simulink model "CaseStudyI_9_Bus"  (R2020a)
settings: Solver=FixedStepAuto  StartTime=0.0  StopTime=Tend  FixedStep=T_s_power  MaxStep=5.0E-5  RelTol=1e-3
values from neighbouring files (symbols this model uses):
  B_s46 = b_s46*Cb    (= 9.5071761847e-07)    [Data_CaseStudyI.m]    (also in Data_CaseStudyII.m; Data_InitialSystem.m)
  B_s54 = b_s54*Cb    (= 1.05902722057e-06)    [Data_CaseStudyI.m]    (also in Data_CaseStudyII.m; Data_InitialSystem.m)
  B_s69 = b_s69*Cb    (= 2.15415764185e-06)    [Data_CaseStudyI.m]    (also in Data_CaseStudyII.m; Data_InitialSystem.m)
  B_s75 = b_s75*Cb    (= 1.84126323577e-06)    [Data_CaseStudyI.m]    (also in Data_CaseStudyII.m; Data_InitialSystem.m)
  B_s87 = b_s87*Cb    (= 8.96562817417e-07)    [Data_CaseStudyI.m]    (also in Data_CaseStudyII.m; Data_InitialSystem.m)
  B_s98 = b_s98*Cb    (= 1.25759482443e-06)    [Data_CaseStudyI.m]    (also in Data_CaseStudyII.m; Data_InitialSystem.m)
  C_dc_DVPP_1_2 = 0.008*(n_DVPP_1_2)    (= 0.8)    [Data_CaseStudyI.m]    (also in Data_CaseStudyII.m)
  C_dc_DVPP_1_3 = 0.008*(n_DVPP_1_3)    (= 0.4)    [Data_CaseStudyI.m]    (also in Data_CaseStudyII.m)
  fb = 50    [Data_CaseStudyI.m]    (also in Data_CaseStudyII.m; Data_InitialSystem.m)
  HGov_dyn = HGov_delay*H_tr_droop    [Data_CaseStudyI.m]    (also in Data_CaseStudyII.m; Data_InitialSystem.m)
  HTurb_tot = H_water_way    [Data_CaseStudyI.m]    (also in Data_CaseStudyII.m; Data_InitialSystem.m)
  I_m_DVPP_1_2 = 2/3*Sb_DVPP_1_2/V_m_DVPP_1_2    [Data_CaseStudyI.m]    (also in Data_CaseStudyII.m)
  I_m_DVPP_1_3 = 2/3*Sb_DVPP_1_3/V_m_DVPP_1_3    [Data_CaseStudyI.m]    (also in Data_CaseStudyII.m)
  i_star_max = 1.3    [Data_CaseStudyI.m]    (also in Data_CaseStudyII.m)
  iabc_DVPP_1_2_0 = T0*idq0_DVPP_1_2    [Data_CaseStudyI.m]    (also in Data_CaseStudyII.m)
  iabc_DVPP_1_3_0 = T0*idq0_DVPP_1_3    [Data_CaseStudyI.m]    (also in Data_CaseStudyII.m)
  K2_DVPP_1 = [-0.0221795494247 -1.60799665656 0.160449825826 -2.94803557381 -11.8081988371 -9.75170960256 0.00463021906909 -49.1667298155]    [ControlGains_DVPP1.mat]
  K3_DVPP_1 = [-0.0591512752956 -1.61493903379 -27.2946107927 -16.2119211358 -14.3657419818 2.05688388773 -2.27328406162 0.146700393037 -150.920793597]    [ControlGains_DVPP1.mat]
  k_dc_DVPP_1_2 = eta_DVPP_1_2/(Vdc_n_DVPP_1_2*m_p_DVPP_1_2)    [Data_CaseStudyI.m]    (also in Data_CaseStudyII.m)
  k_dc_DVPP_1_3 = eta_DVPP_1_3/(Vdc_n_DVPP_1_3*m_p_DVPP_1_3)    [Data_CaseStudyI.m]    (also in Data_CaseStudyII.m)
  ki_i_pu = 1.19    [Data_CaseStudyI.m]    (also in Data_CaseStudyII.m)
  ki_pll = 1700    [Data_CaseStudyI.m]    (also in Data_CaseStudyII.m)
  ki_q_pu = 0.005    [Data_CaseStudyI.m]    (also in Data_CaseStudyII.m)
  kp_i_pu = 0.73    [Data_CaseStudyI.m]    (also in Data_CaseStudyII.m)
  kp_pll = 150    [Data_CaseStudyI.m]    (also in Data_CaseStudyII.m)
  kp_q_pu = 0.05    [Data_CaseStudyI.m]    (also in Data_CaseStudyII.m)
  L1_DVPP_1_2_pu = 0.0186/m_DVPP_1_2    (= 0.000372)    [Data_CaseStudyI.m]    (also in Data_CaseStudyII.m)
  L1_DVPP_1_3_pu = 0.0186/m_DVPP_1_3    (= 0.000744)    [Data_CaseStudyI.m]    (also in Data_CaseStudyII.m)
  l1_MVHV1 = 0    [Data_CaseStudyI.m]    (also in Data_CaseStudyII.m; Data_InitialSystem.m)
  l1_MVHV2 = 0    [Data_CaseStudyI.m]    (also in Data_CaseStudyII.m; Data_InitialSystem.m)
  l1_MVHV3 = 0    [Data_CaseStudyI.m]    (also in Data_CaseStudyII.m; Data_InitialSystem.m)
  L2_DVPP_1_2_pu = L1_DVPP_1_2_pu    (= 0.000372)    [Data_CaseStudyI.m]    (also in Data_CaseStudyII.m)
  L2_DVPP_1_3_pu = L1_DVPP_1_3_pu    (= 0.000744)    [Data_CaseStudyI.m]    (also in Data_CaseStudyII.m)
  l2_MVHV1 = l_s14    (= 0.0576)    [Data_CaseStudyI.m]    (also in Data_CaseStudyII.m; Data_InitialSystem.m)
  l2_MVHV2 = l_s72    (= 0.0625)    [Data_CaseStudyI.m]    (also in Data_CaseStudyII.m; Data_InitialSystem.m)
  l2_MVHV3 = l_s39    (= 0.0586)    [Data_CaseStudyI.m]    (also in Data_CaseStudyII.m; Data_InitialSystem.m)
  l_f_DVPP_1_2 = L_f_DVPP_1_2*w_b/Zb_DVPP_1_2    [Data_CaseStudyI.m]    (also in Data_CaseStudyII.m)
  L_f_DVPP_1_2 = (1/(n_DVPP_1_2))*600*10^-6    (= 6e-06)    [Data_CaseStudyI.m]    (also in Data_CaseStudyII.m)
  l_f_DVPP_1_3 = L_f_DVPP_1_3*w_b/Zb_DVPP_1_3    [Data_CaseStudyI.m]    (also in Data_CaseStudyII.m)
  L_f_DVPP_1_3 = (1/(n_DVPP_1_3))*600*10^-6    (= 1.2e-05)    [Data_CaseStudyI.m]    (also in Data_CaseStudyII.m)
  L_s46 = l_s46*Lb    (= 0.154915055408)    [Data_CaseStudyI.m]    (also in Data_CaseStudyII.m; Data_InitialSystem.m)
  L_s54 = l_s54*Lb    (= 0.143128040323)    [Data_CaseStudyI.m]    (also in Data_CaseStudyII.m; Data_InitialSystem.m)
  L_s69 = l_s69*Lb    (= 0.286256080645)    [Data_CaseStudyI.m]    (also in Data_CaseStudyII.m; Data_InitialSystem.m)
  L_s75 = l_s75*Lb    (= 0.271101346964)    [Data_CaseStudyI.m]    (also in Data_CaseStudyII.m; Data_InitialSystem.m)
  L_s87 = l_s87*Lb    (= 0.12123786945)    [Data_CaseStudyI.m]    (also in Data_CaseStudyII.m; Data_InitialSystem.m)
  L_s98 = l_s98*Lb    (= 0.16973301723)    [Data_CaseStudyI.m]    (also in Data_CaseStudyII.m; Data_InitialSystem.m)
  P_L = pL*Sb    (= 300000000)    [Data_CaseStudyI.m]    (also in Data_CaseStudyII.m; Data_InitialSystem.m)
  p_set_bus1 = P_set_bus1/SbSG1    (= 0.731707317073)    [Data_CaseStudyI.m]    (also in Data_CaseStudyII.m; Data_InitialSystem.m)
  p_set_bus2 = P_set_bus2/SbSG2    (= 0.756707317073)    [Data_CaseStudyI.m]    (also in Data_CaseStudyII.m; Data_InitialSystem.m)
  p_set_bus3 = P_set_bus3/SbSG3    (= 0.731707317073)    [Data_CaseStudyI.m]    (also in Data_CaseStudyII.m; Data_InitialSystem.m)
  pset_DVPP_1_1 = P_set_bus1/SbSG1    (= 0.731707317073)    [Data_CaseStudyI.m]    (also in Data_CaseStudyII.m)
  pset_DVPP_1_2 = 0    [Data_CaseStudyI.m]    (also in Data_CaseStudyII.m)
  pset_DVPP_1_3 = 0    [Data_CaseStudyI.m]    (also in Data_CaseStudyII.m)
  Q_L = qL*Sb    (= 82500000)    [Data_CaseStudyI.m]    (also in Data_CaseStudyII.m; Data_InitialSystem.m)
  qset_DVPP_1_2 = 0    [Data_CaseStudyI.m]    (also in Data_CaseStudyII.m)
  qset_DVPP_1_3 = 0    [Data_CaseStudyI.m]    (also in Data_CaseStudyII.m)
  R1_DVPP_1_2_pu = 0.00734/m_DVPP_1_2    (= 0.0001468)    [Data_CaseStudyI.m]    (also in Data_CaseStudyII.m)
  R1_DVPP_1_3_pu = 0.00734/m_DVPP_1_3    (= 0.0002936)    [Data_CaseStudyI.m]    (also in Data_CaseStudyII.m)
  r1_MVHV1 = 1e-6    (= 1e-06)    [Data_CaseStudyI.m]    (also in Data_CaseStudyII.m; Data_InitialSystem.m)
  r1_MVHV2 = 1e-6    (= 1e-06)    [Data_CaseStudyI.m]    (also in Data_CaseStudyII.m; Data_InitialSystem.m)
  r1_MVHV3 = 1e-6    (= 1e-06)    [Data_CaseStudyI.m]    (also in Data_CaseStudyII.m; Data_InitialSystem.m)
  R2_DVPP_1_2_pu = R1_DVPP_1_2_pu    (= 0.0001468)    [Data_CaseStudyI.m]    (also in Data_CaseStudyII.m)
  R2_DVPP_1_3_pu = R1_DVPP_1_3_pu    (= 0.0002936)    [Data_CaseStudyI.m]    (also in Data_CaseStudyII.m)
  r2_MVHV1 = 1e-6    (= 1e-06)    [Data_CaseStudyI.m]    (also in Data_CaseStudyII.m; Data_InitialSystem.m)
  r2_MVHV2 = 1e-6    (= 1e-06)    [Data_CaseStudyI.m]    (also in Data_CaseStudyII.m; Data_InitialSystem.m)
  r2_MVHV3 = 1e-6    (= 1e-06)    [Data_CaseStudyI.m]    (also in Data_CaseStudyII.m; Data_InitialSystem.m)
  R_dc_DVPP_1_2 = (Vdc_n_DVPP_1_2/(0.05*(Sb_DVPP_1_2)/Vdc_n_DVPP_1_2))    [Data_CaseStudyI.m]    (also in Data_CaseStudyII.m)
  R_dc_DVPP_1_3 = (Vdc_n_DVPP_1_3/(0.05*(Sb_DVPP_1_3)/Vdc_n_DVPP_1_3))    [Data_CaseStudyI.m]    (also in Data_CaseStudyII.m)
  r_f_DVPP_1_2 = R_f_DVPP_1_2/Zb_DVPP_1_2    [Data_CaseStudyI.m]    (also in Data_CaseStudyII.m)
  R_f_DVPP_1_2 = 0.02/n_DVPP_1_2    (= 0.0002)    [Data_CaseStudyI.m]    (also in Data_CaseStudyII.m)
  r_f_DVPP_1_3 = R_f_DVPP_1_3/Zb_DVPP_1_3    [Data_CaseStudyI.m]    (also in Data_CaseStudyII.m)
  R_f_DVPP_1_3 = 0.02/n_DVPP_1_3    (= 0.0004)    [Data_CaseStudyI.m]    (also in Data_CaseStudyII.m)
  R_s46 = r_s46*Zb    (= 8.993)    [Data_CaseStudyI.m]    (also in Data_CaseStudyII.m; Data_InitialSystem.m)
  R_s54 = r_s54*Zb    (= 5.29)    [Data_CaseStudyI.m]    (also in Data_CaseStudyII.m; Data_InitialSystem.m)
  R_s69 = r_s69*Zb    (= 20.631)    [Data_CaseStudyI.m]    (also in Data_CaseStudyII.m; Data_InitialSystem.m)
  R_s75 = r_s75*Zb    (= 16.928)    [Data_CaseStudyI.m]    (also in Data_CaseStudyII.m; Data_InitialSystem.m)
  R_s87 = r_s87*Zb    (= 4.4965)    [Data_CaseStudyI.m]    (also in Data_CaseStudyII.m; Data_InitialSystem.m)
  R_s98 = r_s98*Zb    (= 6.2951)    [Data_CaseStudyI.m]    (also in Data_CaseStudyII.m; Data_InitialSystem.m)
  ReferenceSS2_DVPP_1 = ss(M2T_des_DVPP_1,'minimal')    [Data_CaseStudyI.m]    (also in Data_CaseStudyII.m)
  ReferenceSS3_DVPP_1 = ss(M3T_des_DVPP_1,'minimal')    [Data_CaseStudyI.m]    (also in Data_CaseStudyII.m)
  Rg = 0.03    [Data_CaseStudyI.m]    (also in Data_CaseStudyII.m; Data_InitialSystem.m)
  Sb = 100*10^6    (= 100000000)    [Data_CaseStudyI.m]    (also in Data_CaseStudyII.m; Data_InitialSystem.m)
  Sb_DVPP_1_2 = r_b1*100*10^6*cDVPP_1_2    (= 50000000)    [Data_CaseStudyI.m]    (also in Data_CaseStudyII.m)
  Sb_DVPP_1_3 = r_b1*100*10^6*cDVPP_1_3    (= 25000000)    [Data_CaseStudyI.m]    (also in Data_CaseStudyII.m)
  SbSG1 = r_b1*100*10^6    (= 250000000)    [Data_CaseStudyI.m]    (also in Data_CaseStudyII.m; Data_InitialSystem.m)
  SbSG2 = r_b2*100*10^6    (= 96000000)    [Data_CaseStudyI.m]    (also in Data_CaseStudyII.m; Data_InitialSystem.m)
  SbSG3 = r_b3*100*10^6    (= 64000000)    [Data_CaseStudyI.m]    (also in Data_CaseStudyII.m; Data_InitialSystem.m)
  SGov_dyn = tf([1],[Tg 1])    [Data_CaseStudyI.m]    (also in Data_CaseStudyII.m; Data_InitialSystem.m)
  St_MVHV1 = Sb    (= 100000000)    [Data_CaseStudyI.m]    (also in Data_CaseStudyII.m; Data_InitialSystem.m)
  St_MVHV2 = Sb    (= 100000000)    [Data_CaseStudyI.m]    (also in Data_CaseStudyII.m; Data_InitialSystem.m)
  St_MVHV3 = Sb    (= 100000000)    [Data_CaseStudyI.m]    (also in Data_CaseStudyII.m; Data_InitialSystem.m)
  St_MVLV_DVPP_1_2 = St*m_DVPP_1_2    (= 50000000)    [Data_CaseStudyI.m]    (also in Data_CaseStudyII.m)
  St_MVLV_DVPP_1_3 = St*m_DVPP_1_3    (= 25000000)    [Data_CaseStudyI.m]    (also in Data_CaseStudyII.m)
  STurb_reheat = STurb_ch*STurb_rh    [Data_CaseStudyI.m]    (also in Data_CaseStudyII.m; Data_InitialSystem.m)
  T_load_b3 = 2010    [Data_CaseStudyI.m]    (also in Data_CaseStudyII.m = 1010)
  T_load_b6 = 1010    [Data_CaseStudyI.m]    (also in Data_InitialSystem.m)
  T_s_power = 1e-4    (= 0.0001)    [Data_CaseStudyI.m]    (also in Data_CaseStudyII.m; Data_InitialSystem.m)
  tau_dc_DVPP_1_2 = 0.2    [Data_CaseStudyI.m]    (also in Data_CaseStudyII.m)
  tau_dc_DVPP_1_3 = 0.01    [Data_CaseStudyI.m]    (also in Data_CaseStudyII.m)
  V_m_DVPP_1_2 = VbLV_DVPP_1_2*sqrt(2/3)    [Data_CaseStudyI.m]    (also in Data_CaseStudyII.m)
  V_m_DVPP_1_3 = VbLV_DVPP_1_3*sqrt(2/3)    [Data_CaseStudyI.m]    (also in Data_CaseStudyII.m)
  vabc_DVPP_1_2_0_pu = T0*vdq0_DVPP_1_2_0/V_m_DVPP_1_2    [Data_CaseStudyI.m]    (also in Data_CaseStudyII.m)
  vabc_DVPP_1_3_0_pu = T0*vdq0_DVPP_1_3_0/V_m_DVPP_1_3    [Data_CaseStudyI.m]    (also in Data_CaseStudyII.m)
  VbHV = 230*10^3    (= 230000)    [Data_CaseStudyI.m]    (also in Data_CaseStudyII.m; Data_InitialSystem.m)
  VbLV_DVPP_1_2 = 10^3    (= 1000)    [Data_CaseStudyI.m]    (also in Data_CaseStudyII.m)
  VbLV_DVPP_1_3 = 10^3    (= 1000)    [Data_CaseStudyI.m]    (also in Data_CaseStudyII.m)
  VbMV1 = 16.5*10^3    (= 16500)    [Data_CaseStudyI.m]    (also in Data_CaseStudyII.m; Data_InitialSystem.m)
  VbMV2 = 18.0*10^3    (= 18000)    [Data_CaseStudyI.m]    (also in Data_CaseStudyII.m; Data_InitialSystem.m)
  VbMV3 = 13.8*10^3    (= 13800)    [Data_CaseStudyI.m]    (also in Data_CaseStudyII.m; Data_InitialSystem.m)
  vd0_DVPP_1_2_pu = vd0_DVPP_1_2/V_m_DVPP_1_2    [Data_CaseStudyI.m]    (also in Data_CaseStudyII.m)
  vd0_DVPP_1_3_pu = vd0_DVPP_1_3/V_m_DVPP_1_3    [Data_CaseStudyI.m]    (also in Data_CaseStudyII.m)
  Vdc_n_DVPP_1_2 = 3*V_m_DVPP_1_2    [Data_CaseStudyI.m]    (also in Data_CaseStudyII.m)
  Vdc_n_DVPP_1_3 = 3*V_m_DVPP_1_3    [Data_CaseStudyI.m]    (also in Data_CaseStudyII.m)
  w_b = fb*2*pi    (= 314.159265359)    [Data_CaseStudyI.m]    (also in Data_CaseStudyII.m; Data_InitialSystem.m)
  xid0_DVPP_1_2_pu = 0    [Data_CaseStudyI.m]    (also in Data_CaseStudyII.m)
  xid0_DVPP_1_3_pu = 0    [Data_CaseStudyI.m]    (also in Data_CaseStudyII.m)
  xiq0_DVPP_1_2_pu = 0    [Data_CaseStudyI.m]    (also in Data_CaseStudyII.m)
  xiq0_DVPP_1_3_pu = 0    [Data_CaseStudyI.m]    (also in Data_CaseStudyII.m)
  xpll0_pu = w_b/(ki_pll)    (= 0.184799567858)    [Data_CaseStudyI.m]    (also in Data_CaseStudyII.m)
  xq0_DVPP_1_2_pu = xq0_DVPP_1_2/I_m_DVPP_1_2    [Data_CaseStudyI.m]    (also in Data_CaseStudyII.m)
  ... (+1 more)
undefined symbols (not defined in the file or in its folder): A, B, C, Continuous, Dd, Efd0, gcbh, i_dc, Ka, Kf, p2set, SbSM2, sps_rtmsupport, spsST1AModel, Ta, Tb, Tb1, Tc, Tc1, Tf, VA0, VAmax, VAmin, VImax, VImin, VRmax, VRmin
libraries: powerlib x73, powerlib_meascontrol x16, cstblocks x11, sps_avr x2, simulink_extras x1, simulink x1
(part 1 of 3)
settings Model: SimulationMode=accelerator  Creator=verena  LastModifiedBy=verenahaberle
settings DataIOCC: ExternalInput=getinputstruct(spec1)  FinalStateName=xFinal_c1  InitialState=xInitial_CaseStudyI  LoadInitialState=on  SaveFinalState=on  SaveOperatingPoint=on  SaveFormat=Array  ReturnWorkspaceOutputs=off  TimeSaveName=tout_c1  OutputSaveName=yout_c1  SignalLoggingName=logsout_c1  DSMLoggingName=dsmout_c1
settings OptimizationCC: BlockReduction=off
settings DebuggingCC: UnconnectedInputMsg=none  UnconnectedOutputMsg=none  UnconnectedLineMsg=none  NonCurrentReleaseOperatingPointMsg=warning

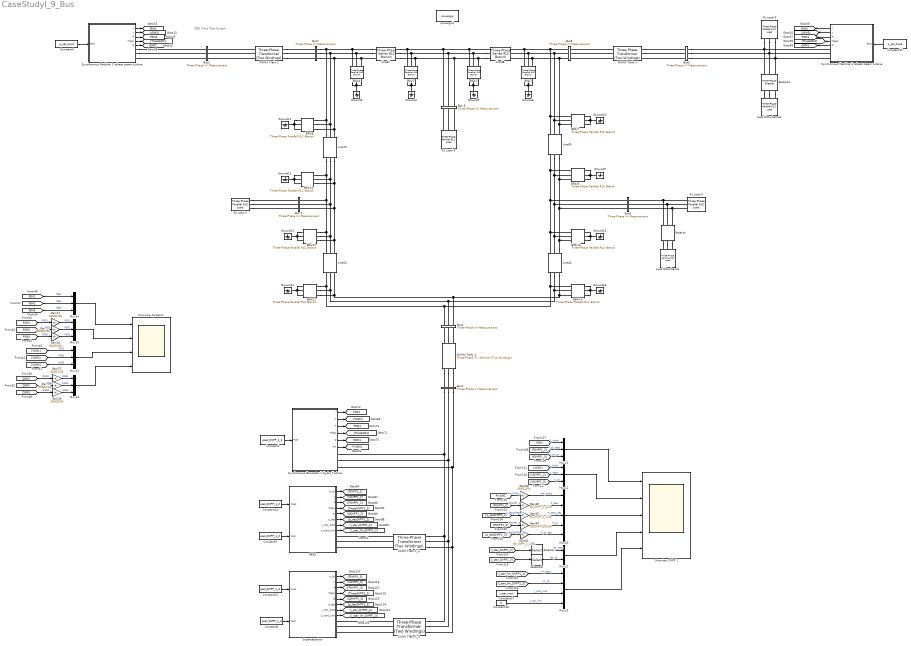
== system CaseStudyI_9_Bus ==
  note: IEEE 9-bus Test System
  B94/1 : powerlib/Elements/Three-Phase Parallel RLC Branch  LConnTagsString=A|B|C  RConnTagsString=A|B|C  BranchType=C  Resistance=1  Inductance=1e-3  Capacitance=B_s98*0.5  Measurements=None
      settings: SourceProductBaseCode=PS
  B94/10 : powerlib/Elements/Three-Phase Parallel RLC Branch  LConnTagsString=A|B|C  RConnTagsString=A|B|C  BranchType=C  Resistance=1  Inductance=1e-3  Capacitance=B_s75*0.5  Measurements=None
      settings: SourceProductBaseCode=PS
  B94/11 : powerlib/Elements/Three-Phase Parallel RLC Branch  LConnTagsString=A|B|C  RConnTagsString=A|B|C  BranchType=C  Resistance=1  Inductance=1e-3  Capacitance=B_s54*0.5  Measurements=None
      settings: SourceProductBaseCode=PS
  B94/12 : powerlib/Elements/Three-Phase Parallel RLC Branch  LConnTagsString=A|B|C  RConnTagsString=A|B|C  BranchType=C  Resistance=1  Inductance=1e-3  Capacitance=B_s54*0.5  Measurements=None
      settings: SourceProductBaseCode=PS
  B94/13 : powerlib/Elements/Three-Phase Parallel RLC Branch  LConnTagsString=A|B|C  RConnTagsString=A|B|C  BranchType=C  Resistance=1  Inductance=1e-3  Capacitance=B_s46*0.5  Measurements=None
      settings: SourceProductBaseCode=PS
  B94/14 : powerlib/Elements/Three-Phase Parallel RLC Branch  LConnTagsString=A|B|C  RConnTagsString=A|B|C  BranchType=C  Resistance=1  Inductance=1e-3  Capacitance=B_s46*0.5  Measurements=None
      settings: SourceProductBaseCode=PS
  B94/2 : powerlib/Elements/Three-Phase Parallel RLC Branch  LConnTagsString=A|B|C  RConnTagsString=A|B|C  BranchType=C  Resistance=1  Inductance=1e-3  Capacitance=B_s87*0.5  Measurements=None
      settings: SourceProductBaseCode=PS
  B94/3 : powerlib/Elements/Three-Phase Parallel RLC Branch  LConnTagsString=A|B|C  RConnTagsString=A|B|C  BranchType=C  Resistance=1  Inductance=1e-3  Capacitance=B_s98*0.5  Measurements=None
      settings: SourceProductBaseCode=PS
  B94/4 : powerlib/Elements/Three-Phase Parallel RLC Branch  LConnTagsString=A|B|C  RConnTagsString=A|B|C  BranchType=C  Resistance=1  Inductance=1e-3  Capacitance=B_s87*0.5  Measurements=None
      settings: SourceProductBaseCode=PS
  B94/7 : powerlib/Elements/Three-Phase Parallel RLC Branch  LConnTagsString=A|B|C  RConnTagsString=A|B|C  BranchType=C  Resistance=1  Inductance=1e-3  Capacitance=B_s69*0.5  Measurements=None
      settings: SourceProductBaseCode=PS
  B94/8 : powerlib/Elements/Three-Phase Parallel RLC Branch  LConnTagsString=A|B|C  RConnTagsString=A|B|C  BranchType=C  Resistance=1  Inductance=1e-3  Capacitance=B_s69*0.5  Measurements=None
      settings: SourceProductBaseCode=PS
  B94/9 : powerlib/Elements/Three-Phase Parallel RLC Branch  LConnTagsString=A|B|C  RConnTagsString=A|B|C  BranchType=C  Resistance=1  Inductance=1e-3  Capacitance=B_s75*0.5  Measurements=None
      settings: SourceProductBaseCode=PS
  BESS : Subsystem
  Breaker : powerlib/Elements/Three-Phase Breaker  InitialState=open  SwitchA=on  SwitchB=on  SwitchC=on  SwitchTimes=[T_load_b6]  External=off  BreakerResistance=0.01  SnubberResistance=1e6  SnubberCapacitance=inf  Measurements=None
  Breaker1 : powerlib/Elements/Three-Phase Breaker  InitialState=open  SwitchA=on  SwitchB=on  SwitchC=on  SwitchTimes=[T_load_b3]  External=off  BreakerResistance=0.01  SnubberResistance=1e6  SnubberCapacitance=inf  Measurements=None
  Bus 5 : powerlib/Measurements/Three-Phase V-I Measurement  VoltageMeasurement=no  SetLabelV=on  LabelV=Vabc_5  Vpu=on  VpuLL=off  CurrentMeasurement=no  SetLabelI=on  LabelI=Iabc_5  Ipu=on  Pbase=S_b  Vbase=V_b  OutputType=Complex  PhasorSimulation=off  PSBequivalent=0
  Bus 8 : powerlib/Measurements/Three-Phase V-I Measurement  VoltageMeasurement=no  SetLabelV=on  LabelV=Vabc_9  Vpu=on  VpuLL=off  CurrentMeasurement=no  SetLabelI=on  LabelI=Iabc_9  Ipu=on  Pbase=S_b  Vbase=V_b  OutputType=Complex  PhasorSimulation=off  PSBequivalent=0
  Bus1 : powerlib/Measurements/Three-Phase V-I Measurement  VoltageMeasurement=phase-to-ground  SetLabelV=on  LabelV=Vabc_B1  Vpu=off  VpuLL=on  CurrentMeasurement=yes  SetLabelI=on  LabelI=Iabc_B1  Ipu=off  Pbase=S_b  Vbase=VbMV1  OutputType=Complex  PhasorSimulation=off  PSBequivalent=0
  Bus2 : powerlib/Measurements/Three-Phase V-I Measurement  VoltageMeasurement=no  SetLabelV=on  LabelV=Vabc_2  Vpu=off  VpuLL=off  CurrentMeasurement=no  SetLabelI=on  LabelI=Iabc_2  Ipu=on  Pbase=Sb  Vbase=VbMV2  OutputType=Complex  PhasorSimulation=off  PSBequivalent=0
  Bus3 : powerlib/Measurements/Three-Phase V-I Measurement  VoltageMeasurement=phase-to-ground  SetLabelV=on  LabelV=Vabc_B3  Vpu=off  VpuLL=on  CurrentMeasurement=yes  SetLabelI=on  LabelI=Iabc_B3  Ipu=off  Pbase=S_b  Vbase=VbMV3  OutputType=Complex  PhasorSimulation=off  PSBequivalent=0
  Bus4 : powerlib/Measurements/Three-Phase V-I Measurement  VoltageMeasurement=no  SetLabelV=off  LabelV=Vabc_6  Vpu=off  VpuLL=off  CurrentMeasurement=no  SetLabelI=off  LabelI=Iabc_6  Ipu=off  Pbase=S_b  Vbase=V_b  OutputType=Complex  PhasorSimulation=off  PSBequivalent=0
  Bus6 : powerlib/Measurements/Three-Phase V-I Measurement  VoltageMeasurement=no  SetLabelV=on  LabelV=Vabc_9  Vpu=on  VpuLL=off  CurrentMeasurement=no  SetLabelI=on  LabelI=Iabc_9  Ipu=on  Pbase=S_b  Vbase=V_b  OutputType=Complex  PhasorSimulation=off  PSBequivalent=0
  Bus7 : powerlib/Measurements/Three-Phase V-I Measurement  VoltageMeasurement=no  SetLabelV=on  LabelV=Vabc_4  Vpu=on  VpuLL=off  CurrentMeasurement=no  SetLabelI=on  LabelI=Iabc_4  Ipu=on  Pbase=S_b  Vbase=V_b  OutputType=Complex  PhasorSimulation=off  PSBequivalent=0
  Bus9 : powerlib/Measurements/Three-Phase V-I Measurement  VoltageMeasurement=phase-to-ground  SetLabelV=on  LabelV=Vabc_9  Vpu=off  VpuLL=off  CurrentMeasurement=yes  SetLabelI=on  LabelI=Iabc_9  Ipu=off  Pbase=S_b  Vbase=V_b  OutputType=Complex  PhasorSimulation=off  PSBequivalent=0
  Constant1 : Constant  Value=pset_DVPP_1_1
  Constant14 : Constant  Value=qset_DVPP_1_2
  Constant15 : Constant  Value=p_set_bus3
  Constant17 : Constant  Value=i_star_max
  Constant18 : Constant  Value=0
  Constant21 : Constant  Value=qset_DVPP_1_3
  Constant4 : Constant  Value=p_set_bus2
  Constant5 : Constant  Value=pset_DVPP_1_2
  Constant6 : Constant  Value=pset_DVPP_1_3
  Gain17 : Gain  Gain=SbSG1/Sb
  Gain18 : Gain  Gain=SbSG2/Sb
  Gain19 : Gain  Gain=SbSG3/Sb
  Gain27 : Gain  Gain=SbSG1/Sb
  Gain28 : Gain  Gain=SbSG2/Sb
  Gain29 : Gain  Gain=SbSG3/Sb
  Gain58 : Gain  Gain=SbSG1/Sb
  Gain59 : Gain  Gain=Sb_DVPP_1_3/Sb
  Gain61 : Gain  Gain=Sb_DVPP_1_3/Sb
  Gain62 : Gain  Gain=Sb_DVPP_1_2/Sb
  Gain65 : Gain  Gain=Sb_DVPP_1_2/Sb
  Ground{3..6,9..16} (12 alike) : powerlib/Elements/Ground  LConnTagsString=a
  LV/MV Trafo 1_2 : powerlib/Elements/Three-Phase Transformer (Two Windings)  Winding1Connection=Yg  Winding2Connection=Yg  CoreType=Three single-phase transformers  SetSaturation=off  Hysteresis=off  DataFile='hysteresis'  SetInitialFlux=off  Measurements=None  UNITS=pu  NominalPower=[St_MVLV_DVPP_1_2, fb]  Winding1=[VbLV_DVPP_1_2,R1_DVPP_1_2_pu,L1_DVPP_1_2_pu]  Winding2=[VbMV1,R2_DVPP_1_2_pu,L2_DVPP_1_2_pu]  Rm=Rm_DVPP_1_2_pu  Lm=Lm_DVPP_1_2_pu  L0=0.5  Saturation=[ 0,0 ; 0.0024,1.2 ; 1.0,1.52 ]  InitialFluxes=[ 0.8 , -0.8 , 0.7 ]  BreakLoop=off  DiscreteSolver=Trapezoidal iterative  DataType=off  TransfoNumber=0
  LV/MV Trafo 1_3 : powerlib/Elements/Three-Phase Transformer (Two Windings)  Winding1Connection=Yg  Winding2Connection=Yg  CoreType=Three single-phase transformers  SetSaturation=off  Hysteresis=off  DataFile='hysteresis'  SetInitialFlux=off  Measurements=None  UNITS=pu  NominalPower=[St_MVLV_DVPP_1_3, fb]  Winding1=[VbLV_DVPP_1_3,R1_DVPP_1_3_pu,L1_DVPP_1_3_pu]  Winding2=[VbMV1,R2_DVPP_1_3_pu,L2_DVPP_1_3_pu]  Rm=Rm_DVPP_1_3_pu  Lm=Lm_DVPP_1_3_pu  L0=0.5  Saturation=[ 0,0 ; 0.0024,1.2 ; 1.0,1.52 ]  InitialFluxes=[ 0.8 , -0.8 , 0.7 ]  BreakLoop=off  DiscreteSolver=Trapezoidal iterative  DataType=off  TransfoNumber=0
  Line46 : powerlib/Elements/Three-Phase Series RLC Branch  LConnTagsString=A|B|C  RConnTagsString=A|B|C  BranchType=RL  Resistance=R_s46  Inductance=L_s46  Capacitance=0  Measurements=None
  Line54 : powerlib/Elements/Three-Phase Series RLC Branch  LConnTagsString=A|B|C  RConnTagsString=A|B|C  BranchType=RL  Resistance=R_s54  Inductance=L_s54  Capacitance=0  Measurements=None
  Line69 : powerlib/Elements/Three-Phase Series RLC Branch  LConnTagsString=A|B|C  RConnTagsString=A|B|C  BranchType=RL  Resistance=R_s69  Inductance=L_s69  Capacitance=0  Measurements=None
  Line75 : powerlib/Elements/Three-Phase Series RLC Branch  LConnTagsString=A|B|C  RConnTagsString=A|B|C  BranchType=RL  Resistance=R_s75  Inductance=L_s75  Capacitance=0  Measurements=None
  Line87 : powerlib/Elements/Three-Phase Series RLC Branch  LConnTagsString=A|B|C  RConnTagsString=A|B|C  BranchType=RL  Resistance=R_s87  Inductance=L_s87  Capacitance=0  Measurements=None
  Line98 : powerlib/Elements/Three-Phase Series RLC Branch  LConnTagsString=A|B|C  RConnTagsString=A|B|C  BranchType=RL  Resistance=R_s98  Inductance=L_s98  Capacitance=0  Measurements=None
  Load Disturbance : powerlib/Elements/Three-Phase Parallel RLC Load  LConnTagsString=A|B|C  Configuration=Y (grounded)  NominalVoltage=VbHV  Vabc=[1e3 1e3 1e3]  Vabcp=[1e3 1e3 1e3]  NominalFrequency=fb  UnbalancedPower=off  ActivePower=Load_step_b6  InductivePower=0  CapacitivePower=0  Pabc=[10e3 9e3 11e3]  QLabc=[100 90 110]  QCabc=[100 90 110]  Pabcp=[10e3 9e3 11e3]  QLabcp=[100 90 110]  QCabcp=[100 90 110]  Measurements=None  LoadType=constant Z
  Load Disturbance1 : powerlib/Elements/Three-Phase Parallel RLC Load  LConnTagsString=A|B|C  Configuration=Y (grounded)  NominalVoltage=VbMV3  Vabc=[1e3 1e3 1e3]  Vabcp=[1e3 1e3 1e3]  NominalFrequency=fb  UnbalancedPower=off  ActivePower=Load_step_b3  InductivePower=0  CapacitivePower=0  Pabc=[10e3 9e3 11e3]  QLabc=[100 90 110]  QCabc=[100 90 110]  Pabcp=[10e3 9e3 11e3]  QLabcp=[100 90 110]  QCabcp=[100 90 110]  Measurements=None  LoadType=constant Z
  "MV/HV Trafo 1 " : powerlib/Elements/Three-Phase Transformer (Two Windings)  Winding1Connection=Yg  Winding2Connection=Yg  CoreType=Three single-phase transformers  SetSaturation=off  Hysteresis=off  DataFile='hysteresis'  SetInitialFlux=off  Measurements=None  UNITS=pu  NominalPower=[St_MVHV1 fb ]  Winding1=[VbMV1 r1_MVHV1 l1_MVHV1]  Winding2=[VbHV r2_MVHV1 l2_MVHV1]  Rm=500  Lm=500  L0=0.5  Saturation="[ 0,0  ;  0.005,1.2  ;  1.0,1.4 ]"  InitialFluxes=[ 0.8 , -0.8 , 0.7 ]  BreakLoop=off  DiscreteSolver=Backward Euler robust  DataType=off  TransfoNumber=0
  "MV/HV Trafo 2 " : powerlib/Elements/Three-Phase Transformer (Two Windings)  Winding1Connection=Yg  Winding2Connection=Yg  CoreType=Three single-phase transformers  SetSaturation=off  Hysteresis=off  DataFile='hysteresis'  SetInitialFlux=off  Measurements=None  UNITS=pu  NominalPower=[St_MVHV2 fb ]  Winding1=[VbMV2 r1_MVHV2 l1_MVHV2]  Winding2=[ VbHV r2_MVHV2 l2_MVHV2]  Rm=500  Lm=500  L0=0.5  Saturation="[ 0,0  ;  0.005,1.2  ;  1.0,1.4 ]"  InitialFluxes=[ 0.8 , -0.8 , 0.7 ]  BreakLoop=off  DiscreteSolver=Backward Euler robust  DataType=off  TransfoNumber=0
  "MV/HV Trafo 3 " : powerlib/Elements/Three-Phase Transformer (Two Windings)  Winding1Connection=Yg  Winding2Connection=Yg  CoreType=Three single-phase transformers  SetSaturation=off  Hysteresis=off  DataFile='hysteresis'  SetInitialFlux=off  Measurements=None  UNITS=pu  NominalPower=[St_MVHV3 fb ]  Winding1=[VbMV3 r1_MVHV3 l1_MVHV3]  Winding2=[ VbHV r2_MVHV3 l2_MVHV3]  Rm=500  Lm=500  L0=0.5  Saturation="[ 0,0  ;  0.005,1.2  ;  1.0,1.4 ]"  InitialFluxes=[ 0.8 , -0.8 , 0.7 ]  BreakLoop=off  DiscreteSolver=Backward Euler robust  DataType=off  TransfoNumber=0
  Mux{10..14,21} (6 alike) : Mux  Inputs=3
  Mux20 : Mux  Inputs=5
  Mux22 : Mux  Inputs=2
  Mux23 : Mux
  Overview DVPP 1 : Scope  NumInputPorts=5
  Overview System1 : Scope  NumInputPorts=4
  RL Load 3 : powerlib/Elements/Three-Phase Parallel RLC Load  LConnTagsString=A|B|C  Configuration=Y (grounded)  NominalVoltage=VbMV3  Vabc=[1e3 1e3 1e3]  Vabcp=[1e3 1e3 1e3]  NominalFrequency=fb  UnbalancedPower=off  ActivePower=P_L/12  InductivePower=Q_L/12  CapacitivePower=0  Pabc=[10e3 9e3 11e3]  QLabc=[100 90 110]  QCabc=[100 90 110]  Pabcp=[10e3 9e3 11e3]  QLabcp=[100 90 110]  QCabcp=[100 90 110]  Measurements=None  LoadType=constant Z
  RL Load 5 : powerlib/Elements/Three-Phase Parallel RLC Load  LConnTagsString=A|B|C  Configuration=Y (grounded)  NominalVoltage=VbHV  Vabc=[1e3 1e3 1e3]  Vabcp=[1e3 1e3 1e3]  NominalFrequency=fb  UnbalancedPower=off  ActivePower=P_L/3  InductivePower=Q_L/3  CapacitivePower=0  Pabc=[10e3 9e3 11e3]  QLabc=[100 90 110]  QCabc=[100 90 110]  Pabcp=[10e3 9e3 11e3]  QLabcp=[100 90 110]  QCabcp=[100 90 110]  Measurements=None  LoadType=constant Z
  RL Load 6 : powerlib/Elements/Three-Phase Parallel RLC Load  LConnTagsString=A|B|C  Configuration=Y (grounded)  NominalVoltage=VbHV  Vabc=[1e3 1e3 1e3]  Vabcp=[1e3 1e3 1e3]  NominalFrequency=fb  UnbalancedPower=off  ActivePower=P_L/3  InductivePower=Q_L/3  CapacitivePower=0  Pabc=[10e3 9e3 11e3]  QLabc=[100 90 110]  QCabc=[100 90 110]  Pabcp=[10e3 9e3 11e3]  QLabcp=[100 90 110]  QCabcp=[100 90 110]  Measurements=None  LoadType=constant Z
  "RL Load 8 " : powerlib/Elements/Three-Phase Parallel RLC Load  LConnTagsString=A|B|C  Configuration=Y (grounded)  NominalVoltage=VbHV  Vabc=[1e3 1e3 1e3]  Vabcp=[1e3 1e3 1e3]  NominalFrequency=fb  UnbalancedPower=off  ActivePower=P_L/4  InductivePower=Q_L/4  CapacitivePower=0  Pabc=[10e3 9e3 11e3]  QLabc=[100 90 110]  QCabc=[100 90 110]  Pabcp=[10e3 9e3 11e3]  QLabcp=[100 90 110]  QCabcp=[100 90 110]  Measurements=None  LoadType=constant Z
  Selector7 : Selector  InputPortWidth=3  IndexOptions=Index vector (dialog)  Indices=[1]  OutputSizes=1
  Selector8 : Selector  InputPortWidth=3  IndexOptions=Index vector (dialog)  Indices=[1]  OutputSizes=1
  Supercapacitor : Subsystem
  Synchronous Generator 1 Hydro Turbine : Subsystem
  Synchronous Machine 2 reheat steam turbine : Subsystem
  Synchronous Machine 3 reheat steam turbine : Subsystem
  powergui1 : powerlib/powergui  Priority=1  SimulationMode=Discrete  SampleTime=T_s_power  frequency=fb  Iterations=100  frequencyindice=0  Pbase=100e6  ErrMax=0.0001  UnitsV=kV  UnitsW=MW  buscounter=3  FunctionMessages=off  echomessages=off  EnableUseOfTLC=off  CurrentSourceSwitches=off  DisableSnubberDevices=off  DisableRonSwitches=off  DisableVfSwitches=off  DisplayEquations=off  AutomaticDiscreteSolvers=off  SolverType=Tustin/Backward Euler (TBE)  Interpol=off  ExternalGateDelay=off  methode=off  Ts=100  x0status=blocks  SPID=off  SwTol=0  HookPort=off  NonlinearTolerance=1e-5  nMaxIteration=200  ContinueOnMaxIteration=off  RestoreLinks=warning  ResistiveCurrentMeasurement=off  Frange=[0:2:500]  Ylog=off  Xlog=on  ShowGrid=off  save=off  variable=ZData  structure=0  ZoomFFT=off  StartTime=0.0  cycles=1  DisplayStyle=1  fundamental=60  FreqAxis=off  MaxFrequency=1000  frequencyindicesteady=1  RmsSteady=1  display=off
  tag scope: PSM1=global, PSM2=global, PSM3=global, PmSM1=global, QSM1=global, QSM2=global, QSM3=global, fSM1=global, fSM2=global, fSM3=global
  wires:
  Constant4/1 -> Synchronous Machine 2 reheat steam turbine/1(Pset)
  Synchronous Machine 2 reheat steam turbine/1(f) -> [fSM2]
  Synchronous Machine 2 reheat steam turbine/2(V) -> [VSM2]
  Synchronous Machine 2 reheat steam turbine/3(P) -> [PSM2]
  Synchronous Machine 2 reheat steam turbine/4(Theta) -> [ThetaSM2]
  Synchronous Machine 2 reheat steam turbine/5(Q) -> [QSM2]
  Synchronous Machine 3 reheat steam turbine/4(Theta) -> [ThetaSM3]
  Synchronous Machine 3 reheat steam turbine/2(V) -> [VSM3]
  Synchronous Machine 3 reheat steam turbine/3(P) -> [PSM3]
  Constant15/1 -> Synchronous Machine 3 reheat steam turbine/1(Pset)
  Synchronous Machine 3 reheat steam turbine/1(f) -> [fSM3]
  Synchronous Machine 3 reheat steam turbine/5(Q) -> [QSM3]
  Constant18/1 -> Mux23/4  "i_star_min"
  Supercapacitor/6(p_des) -> [p_desDVPP1_3]
  Mux21/1 -> Overview DVPP 1/1
  [i_star_lim_DVPP1_3] -> Mux23/2  "|i*_sc|"
  Constant21/1 -> Supercapacitor/1(Qset)
  Mux11/1 -> Overview DVPP 1/2
  Mux22/1 -> Overview DVPP 1/4
  Mux20/1 -> Overview DVPP 1/3
  Synchronous Generator 1 Hydro Turbine/2(V) -> [VSM1]
  Constant1/1 -> Synchronous Generator 1 Hydro Turbine/1(Pset)
  Gain58/1 -> Mux20/1  "Pm_hydro"
  Supercapacitor/8(|i_star3_lim|) -> [i_star_lim_DVPP1_3]
  [PmSM1] -> Gain58/1  "PmDVPP1_1"
  Constant6/1 -> Supercapacitor/2(Pset)
  [p_desDVPP1_2] -> Gain62/1  "p_desDVPP1_2"
  Supercapacitor/2(V) -> [VDVPP1_3]
  [i_star_DVPP1_3] -> Selector8/1
  [fDVPP1_3] -> Mux21/3  "f_pll_sc"
  [p_desDVPP1_3] -> Gain61/1  "p_desDVPP1_3"
  Mux23/1 -> Overview DVPP 1/5
  [PDVPP1_2] -> Gain65/1  "PDVPP1_2"
  [i_star_DVPP1_2] -> Selector7/1
  Supercapacitor/4(Theta) -> [ThetaDVPP1_3]
  Synchronous Generator 1 Hydro Turbine/6(Pm) -> [PmSM1]
  Supercapacitor/5(Q) -> [QDVPP1_3]
  Constant17/1 -> Mux23/3  "i_star_max"
  Constant5/1 -> BESS/2(Pset)
  Supercapacitor/1(w_pll) -> [fDVPP1_3]
  Synchronous Generator 1 Hydro Turbine/4(Theta) -> [ThetaSM1]
  [VDVPP1_2] -> Mux11/2  "V_bess"
  [VDVPP1_3] -> Mux11/3  "V_sc"
  BESS/7(i_star_dq01) -> [i_star_DVPP1_2]
  BESS/3(P) -> [PDVPP1_2]
  Supercapacitor/3(P) -> [PDVPP1_3]
  BESS/6(p_des) -> [p_desDVPP1_2]
  Synchronous Generator 1 Hydro Turbine/3(P) -> [PSM1]
  [PDVPP1_3] -> Gain59/1  "PDVPP1_3"
  Supercapacitor/7(i_star_dq01) -> [i_star_DVPP1_3]
  BESS/8(|i_star3_lim|) -> [i_star_lim_DVPP1_2]
  Synchronous Generator 1 Hydro Turbine/5(Q) -> [QSM1]
  [fSM1] -> Mux21/1  "f_hydro"
  Synchronous Generator 1 Hydro Turbine/1(f) -> [fSM1]
  [fDVPP1_2] -> Mux21/2  "f_pll_bess"
  Selector7/1 -> Mux22/1  "id*_bess"
  BESS/2(V) -> [VDVPP1_2]
  BESS/1(w_pll) -> [fDVPP1_2]
  Selector8/1 -> Mux22/2  "id*_sc"
  [VSM1] -> Mux11/1  "V_hydro"
  Constant14/1 -> BESS/1(Qset)
  BESS/5(Q) -> [QDVPP1_2]
  BESS/4(Theta) -> [ThetaDVPP1_2]
  [i_star_lim_DVPP1_2] -> Mux23/1  "|i*_bess|"
  [VSM1] -> Mux12/1  "VSG1"
  [fSM3] -> Mux14/3  "fSG3"
  [PSM2] -> Gain18/1  "PSG2"
  [QSM1] -> Gain27/1  "QSG1"
  Mux14/1 -> Overview System1/1
  Gain28/1 -> Mux13/2  "QSG2"
  [VSM2] -> Mux12/2  "VSG2"
  [QSM2] -> Gain28/1  "QSG2"
  [PSM3] -> Gain19/1  "PSG3"
  Mux13/1 -> Overview System1/4
  Mux12/1 -> Overview System1/3
  Gain27/1 -> Mux13/1  "QSG1"
  Gain19/1 -> Mux10/3  "PSG3"
  [QSM3] -> Gain29/1  "QSG3"
  Gain18/1 -> Mux10/2  "PSG2"
  Gain17/1 -> Mux10/1  "PSG1"
  Gain29/1 -> Mux13/3  "QSG3"
  [fSM2] -> Mux14/2  "fSG2"
  [PSM1] -> Gain17/1  "PSG1"
  [fSM1] -> Mux14/1  "fSG1"
  Mux10/1 -> Overview System1/2
  [VSM3] -> Mux12/3  "VSG3"
  Gain65/1 -> Mux20/2  "P_bess"
  Gain62/1 -> Mux20/3  "P_bess_des"
  Gain59/1 -> Mux20/4  "P_sc"
  Gain61/1 -> Mux20/5  "P_sc_des"
  connections:
  B94/1/RConn1 -- Ground6/LConn1 -- B94/1/RConn2 -- B94/1/RConn3
  B94/9/RConn1 -- Ground11/LConn1 -- B94/9/RConn3 -- B94/9/RConn2
  RL Load 6/LConn3 -- Breaker/RConn3 -- Bus6/LConn3
  Bus 5/LConn1 -- Line54/LConn1 -- B94/12/LConn1 -- Line75/RConn1 -- B94/10/LConn1
  "MV/HV Trafo 2 "/RConn1 -- Bus7/RConn1
  "MV/HV Trafo 1 "/LConn1 -- Bus1/LConn1
  B94/3/RConn3 -- B94/3/RConn1 -- B94/3/RConn2 -- Ground5/LConn1
  B94/10/LConn3 -- Line75/RConn3 -- Line54/LConn3 -- B94/12/LConn3 -- Bus 5/LConn3
  B94/13/LConn1 -- Line46/LConn1 -- Bus6/RConn1 -- B94/8/LConn1 -- Line69/RConn1
  B94/8/LConn2 -- B94/13/LConn2 -- Line46/LConn2 -- Bus6/RConn2 -- Line69/RConn2
  Ground16/LConn1 -- B94/14/RConn3 -- B94/14/RConn1 -- B94/14/RConn2
  B94/11/RConn2 -- Ground14/LConn1 -- B94/11/RConn3 -- B94/11/RConn1
  Line87/LConn2 -- B94/4/LConn2 -- Bus7/LConn2 -- Line75/LConn2 -- B94/9/LConn2
  B94/2/RConn1 -- Ground4/LConn1 -- B94/2/RConn2 -- B94/2/RConn3
  "MV/HV Trafo 3 "/LConn1 -- Bus3/LConn1
  Line98/LConn2 -- B94/3/LConn2 -- Bus 8/RConn2 -- B94/2/LConn2 -- Line87/RConn2
  Line98/RConn2 -- B94/1/LConn2 -- B94/7/LConn2 -- Line69/LConn2 -- Bus9/RConn2
  Line98/LConn3 -- B94/3/LConn3 -- Bus 8/RConn1 -- Line87/RConn3 -- B94/2/LConn3
  RL Load 6/LConn1 -- Breaker/RConn1 -- Bus6/LConn1
  B94/11/LConn2 -- Line54/RConn2 -- Line46/RConn2 -- B94/14/LConn2 -- Bus4/LConn2
  Ground12/LConn1 -- B94/10/RConn3 -- B94/10/RConn1 -- B94/10/RConn2
  B94/14/LConn3 -- Line46/RConn3 -- Bus4/LConn3 -- B94/11/LConn3 -- Line54/RConn3
  Line54/RConn1 -- B94/11/LConn1 -- Bus4/LConn1 -- Line46/RConn1 -- B94/14/LConn1
  "MV/HV Trafo 3 "/RConn1 -- Bus9/LConn1
  B94/2/LConn1 -- Line87/RConn1 -- Bus 8/RConn3 -- B94/3/LConn1 -- Line98/LConn1
  Line98/RConn3 -- B94/1/LConn3 -- Bus9/RConn3 -- B94/7/LConn3 -- Line69/LConn3
  Line87/LConn3 -- B94/4/LConn3 -- Bus7/LConn3 -- B94/9/LConn3 -- Line75/LConn3
  Line46/LConn3 -- B94/8/LConn3 -- Line69/RConn3 -- Bus6/RConn3 -- B94/13/LConn3
  "MV/HV Trafo 2 "/LConn1 -- Bus2/LConn1
  B94/8/RConn3 -- B94/8/RConn1 -- B94/8/RConn2 -- Ground9/LConn1
  Line98/RConn1 -- B94/1/LConn1 -- Bus9/RConn1 -- B94/7/LConn1 -- Line69/LConn1
  B94/10/LConn2 -- Line75/RConn2 -- Line54/LConn2 -- B94/12/LConn2 -- Bus 5/LConn2
  B94/4/RConn3 -- B94/4/RConn1 -- B94/4/RConn2 -- Ground3/LConn1
  Line87/LConn1 -- B94/4/LConn1 -- B94/9/LConn1 -- Line75/LConn1 -- Bus7/LConn1
  B94/7/RConn1 -- Ground10/LConn1 -- B94/7/RConn3 -- B94/7/RConn2
  B94/12/RConn1 -- Ground13/LConn1 -- B94/12/RConn3 -- B94/12/RConn2
  RL Load 6/LConn2 -- Breaker/RConn2 -- Bus6/LConn2
  B94/13/RConn1 -- Ground15/LConn1 -- B94/13/RConn3 -- B94/13/RConn2
  Synchronous Machine 2 reheat steam turbine/RConn3 -- Bus2/RConn3
  "RL Load 8 "/LConn3 -- Bus 8/LConn1
  "MV/HV Trafo 3 "/LConn2 -- Bus3/LConn2
  "MV/HV Trafo 3 "/RConn2 -- Bus9/LConn2
  "MV/HV Trafo 1 "/LConn3 -- Bus1/LConn3
  "MV/HV Trafo 1 "/RConn1 -- Bus4/RConn1
  "MV/HV Trafo 2 "/RConn3 -- Bus7/RConn3
  RL Load 5/LConn2 -- Bus 5/RConn2
  "MV/HV Trafo 2 "/RConn2 -- Bus7/RConn2
  "MV/HV Trafo 1 "/RConn2 -- Bus4/RConn2
  "RL Load 8 "/LConn2 -- Bus 8/LConn2
  "MV/HV Trafo 2 "/LConn2 -- Bus2/LConn2
  RL Load 5/LConn3 -- Bus 5/RConn3
  "RL Load 8 "/LConn1 -- Bus 8/LConn3
  Synchronous Machine 2 reheat steam turbine/RConn1 -- Bus2/RConn1
  "MV/HV Trafo 2 "/LConn3 -- Bus2/LConn3
  "MV/HV Trafo 1 "/LConn2 -- Bus1/LConn2
  "MV/HV Trafo 3 "/RConn3 -- Bus9/LConn3
  RL Load 5/LConn1 -- Bus 5/RConn1
  Synchronous Machine 2 reheat steam turbine/RConn2 -- Bus2/RConn2
  "MV/HV Trafo 1 "/RConn3 -- Bus4/RConn3
  Bus3/LConn3 -- "MV/HV Trafo 3 "/LConn3
  RL Load 3/LConn3 -- Breaker1/RConn3 -- Synchronous Machine 3 reheat steam turbine/RConn3 -- Bus3/RConn3
  LV/MV Trafo 1_3/RConn2 -- Bus1/RConn2 -- Synchronous Generator 1 Hydro Turbine/RConn2 -- LV/MV Trafo 1_2/RConn2
  LV/MV Trafo 1_3/RConn3 -- LV/MV Trafo 1_2/RConn3 -- Bus1/RConn3 -- Synchronous Generator 1 Hydro Turbine/RConn3
  LV/MV Trafo 1_3/RConn1 -- Bus1/RConn1 -- Synchronous Generator 1 Hydro Turbine/RConn1 -- LV/MV Trafo 1_2/RConn1
  LV/MV Trafo 1_2/LConn1 -- BESS/RConn1
  LV/MV Trafo 1_2/LConn3 -- BESS/RConn3
  Supercapacitor/RConn1 -- LV/MV Trafo 1_3/LConn1
  LV/MV Trafo 1_3/LConn2 -- Supercapacitor/RConn2
  LV/MV Trafo 1_2/LConn2 -- BESS/RConn2
  LV/MV Trafo 1_3/LConn3 -- Supercapacitor/RConn3
  Breaker/LConn3 -- Load Disturbance/LConn3
  Breaker/LConn1 -- Load Disturbance/LConn1
  Breaker/LConn2 -- Load Disturbance/LConn2
  RL Load 3/LConn2 -- Breaker1/RConn2 -- Synchronous Machine 3 reheat steam turbine/RConn2 -- Bus3/RConn2
  Bus3/RConn1 -- Breaker1/RConn1 -- Synchronous Machine 3 reheat steam turbine/RConn1 -- RL Load 3/LConn1
  Breaker1/LConn1 -- Load Disturbance1/LConn1
  Breaker1/LConn2 -- Load Disturbance1/LConn2
  Breaker1/LConn3 -- Load Disturbance1/LConn3

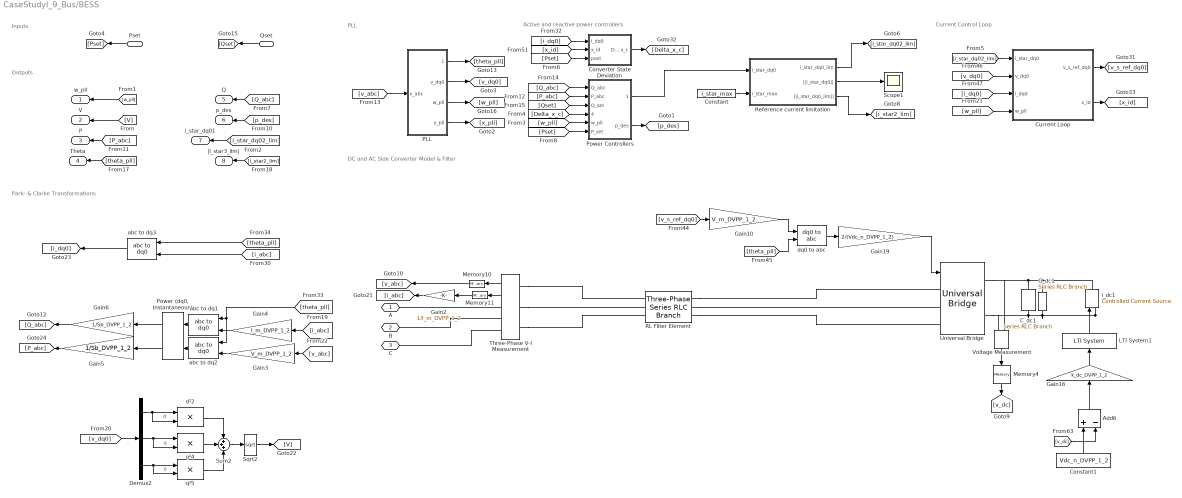
== system CaseStudyI_9_Bus/BESS ==
  note: Inputs
  note: Active and reactive power controllers
  note: PLL
  note: Outputs
  note: Current Control Loop
  note: Park- & Clarke Transformations
  note: DC and AC Side Converter Model & Filter
  Qset : Inport
  Pset : Inport  Port=2
  Add6 : Sum  Inputs=+-
  C_dc1 : powerlib/Elements/Series RLC Branch  LConnTagsString=__new0  RConnTagsString=__new0  BranchType=C  Resistance=1  Inductance=1e-3  SetiL0=off  InitialCurrent=0  Capacitance=C_dc_DVPP_1_2  Setx0=off  InitialVoltage=Vdc_n  Measurements=None
  Constant : Constant  Value=i_star_max
  Constant1 : Constant  Value=Vdc_n_DVPP_1_2
  Converter State Deviation : Subsystem
  Current Loop : Subsystem  AncestorBlock=Library/Grid-Forming Converter Controlled by Droop Control /Current Loop
  Demux2 : Demux  Outputs=3
  G_dc1 : powerlib/Elements/Series RLC Branch  LConnTagsString=__new0  RConnTagsString=__new0  BranchType=R  Resistance=R_dc_DVPP_1_2  Inductance=1e-3  SetiL0=off  InitialCurrent=0  Capacitance=1e-6  Setx0=off  InitialVoltage=0  Measurements=None
  Gain10 : Gain  Gain=V_m_DVPP_1_2
  Gain16 : Gain  Gain=k_dc_DVPP_1_2
  Gain19 : Gain  Gain=2/(Vdc_n_DVPP_1_2)
  Gain2 : Gain  Gain=1/I_m_DVPP_1_2
  Gain3 : Gain  Gain=V_m_DVPP_1_2
  Gain4 : Gain  Gain=I_m_DVPP_1_2
  Gain5 : Gain  Gain=1/Sb_DVPP_1_2
  Gain6 : Gain  Gain=1/Sb_DVPP_1_2
  LTI System1 : cstblocks/LTI System  sys=tf(1,[tau_dc_DVPP_1_2 1])  IC=[]
  Memory10 : Memory  InitialCondition=[vabc_DVPP_1_2_0_pu(1), vabc_DVPP_1_2_0_pu(2), vabc_DVPP_1_2_0_pu(3)]
  Memory11 : Memory  InitialCondition=[iabc_DVPP_1_2_0(1), iabc_DVPP_1_2_0(2), iabc_DVPP_1_2_0(3)]
  Memory4 : Memory
  PLL : Subsystem
  "Power (dq0, Instantaneous)" : powerlib_meascontrol/Measurements/Power (dq0, Instantaneous)
      settings: SourceProductBaseCode=PS
  Power Controllers : Subsystem
  RL Filter Element : powerlib/Elements/Three-Phase Series RLC Branch  LConnTagsString=A|B|C  RConnTagsString=A|B|C  BranchType=RL  Resistance=R_f_DVPP_1_2  Inductance=L_f_DVPP_1_2  Capacitance=0  Measurements=Branch currents
  Reference current limitation : Subsystem
  Scope1 : Scope
  Sqrt2 : Sqrt  SaturateOnIntegerOverflow=on
  Sum2 : Sum  Inputs=+++  InputSameDT=on  SaturateOnIntegerOverflow=on  OutDataTypeStr=Inherit: Same as first input
  Three-Phase V-I Measurement : powerlib/Measurements/Three-Phase V-I Measurement  VoltageMeasurement=phase-to-ground  SetLabelV=off  LabelV=Vabc  Vpu=on  VpuLL=off  CurrentMeasurement=yes  SetLabelI=off  LabelI=Iabc  Ipu=off  Pbase=Sb_conv  Vbase=VbLV_DVPP_1_2  OutputType=Complex  PhasorSimulation=off  PSBequivalent=0
  Universal Bridge : powerlib/Power Electronics/Universal Bridge  Arms=3  SnubberResistance=1e5  SnubberCapacitance=inf  Device=Average-model based VSC  Ron=1e-3  Lon=0  ForwardVoltages="[  0  0  ]"  ForwardVoltage=0  GTOparameters=[ 10e-6 , 20e-6 ]  IGBTparameters=[ 1e-6 , 2e-6 ]  Measurements=None  Measurements_2=None  converterType=Rectifier
  Voltage Measurement : powerlib/Measurements/Voltage Measurement  PhasorSimulation=off  OutputType=Complex  PSBequivalent=0
  abc to dq1 : powerlib_meascontrol/Transformations/abc to dq0  Alignment=90 degrees behind phase A axis
  abc to dq2 : powerlib_meascontrol/Transformations/abc to dq0  Alignment=90 degrees behind phase A axis
  abc to dq3 : powerlib_meascontrol/Transformations/abc to dq0  Alignment=90 degrees behind phase A axis
  dq0 to abc : powerlib_meascontrol/Transformations/dq0 to abc  Alignment=90 degrees behind phase A axis
  d²2 : Product  InputSameDT=on  RndMeth=Zero  SaturateOnIntegerOverflow=on  OutDataTypeStr=Inherit: Same as first input
  i_dc1 : powerlib/Electrical Sources/Controlled Current Source  Initialize=off  Source_Type=DC  Amplitude=i_dc  Phase=0  Frequency=0  Measurements=None
  q²4 : Product  InputSameDT=on  RndMeth=Zero  SaturateOnIntegerOverflow=on  OutDataTypeStr=Inherit: Same as first input
  q²5 : Product  InputSameDT=on  RndMeth=Zero  SaturateOnIntegerOverflow=on  OutDataTypeStr=Inherit: Same as first input
  A : PMIOPort  Side=Right
  B : PMIOPort  Port=2  Side=Right
  C : PMIOPort  Port=3  Side=Right
  w_pll : Outport  VectorParamsAs1DForOutWhenUnconnected=off
  V : Outport  Port=2  VectorParamsAs1DForOutWhenUnconnected=off
  P : Outport  Port=3  VectorParamsAs1DForOutWhenUnconnected=off
  Theta : Outport  Port=4  VectorParamsAs1DForOutWhenUnconnected=off
  Q : Outport  Port=5  VectorParamsAs1DForOutWhenUnconnected=off
  p_des : Outport  Port=6  VectorParamsAs1DForOutWhenUnconnected=off
  i_star_dq01 : Outport  Port=7  VectorParamsAs1DForOutWhenUnconnected=off
  |i_star3_lim| : Outport  Port=8  VectorParamsAs1DForOutWhenUnconnected=off
  wires:
  PLL/4(x_pll) -> [x_pll]
  [v_abc] -> PLL/1(v_abc)
  [i_star_dq02_lim] -> i_star_dq01/1
  PLL/2(v_dq0) -> [v_dq0]
  [p_des] -> p_des/1
  PLL/1(theta_pll) -> [theta_pll]
  PLL/3(w_pll) -> [w_pll]
  [V] -> V/1
  [w_pll] -> w_pll/1
  [theta_pll] -> Theta/1
  Power Controllers/2(p_des) -> [p_des]
  Power Controllers/1(i_star_dq0) -> Reference current limitation/1(i_star_dq0)
  [Q_abc] -> Q/1
  Qset/1 -> [Qset]
  [P_abc] -> P/1
  Constant/1 -> Reference current limitation/2(i_star_max)
  Reference current limitation/2(||i_star_dq0||) -> Scope1/1
  [i_star2_lim] -> |i_star3_lim|/1
  [w_pll] -> Current Loop/4(w_pll)
  [i_dq0] -> Current Loop/3(i_dq0)
  Reference current limitation/1(i_star_dq0_lim) -> [i_star_dq02_lim]
  [v_dq0] -> Current Loop/2(v_dq0)
  [v_dq0] -> Demux2/1
  Sum2/1 -> Sqrt2/1
  [i_abc] -> Gain4/1
  Demux2/3 -> q²5/2, q²5/1  "0"
  Demux2/1 -> d²2/1, d²2/2  "d"
  abc to dq1/1 -> "Power (dq0, Instantaneous)"/2
  Gain5/1 -> [P_abc]
  Gain4/1 -> abc to dq1/1
  Gain3/1 -> abc to dq2/1
  q²4/1 -> Sum2/2
  Gain6/1 -> [Q_abc]
  Gain19/1 -> Universal Bridge/1
  Add6/1 -> Gain16/1
  [v_abc] -> Gain3/1
  [theta_pll] -> abc to dq3/2
  Voltage Measurement/1 -> Memory4/1
  d²2/1 -> Sum2/1
  [theta_pll] -> abc to dq2/2, abc to dq1/2
  dq0 to abc/1 -> Gain19/1
  Three-Phase V-I Measurement/1 -> Memory10/1
  "Power (dq0, Instantaneous)"/2 -> Gain6/1
  Sqrt2/1 -> [V]
  "Power (dq0, Instantaneous)"/1 -> Gain5/1
  Demux2/2 -> q²4/1, q²4/2  "q"
  [v_dc] -> Add6/2
  q²5/1 -> Sum2/3
  abc to dq2/1 -> "Power (dq0, Instantaneous)"/1
  Memory4/1 -> [v_dc]
  LTI System1/1 -> i_dc1/1
  Gain10/1 -> dq0 to abc/1
  [theta_pll] -> dq0 to abc/2
  [i_abc] -> abc to dq3/1
  [v_s_ref_dq0] -> Gain10/1
  Gain16/1 -> LTI System1/1
  Constant1/1 -> Add6/1
  Converter State Deviation/1(Delta x_c) -> [Delta_x_c]
  Current Loop/2(x_id) -> [x_id]
  Current Loop/1(v_s_ref_dq0) -> [v_s_ref_dq0]
  [P_abc] -> Power Controllers/2(P_abc)
  [Delta_x_c] -> Power Controllers/4(Delta x_c)
  [Q_abc] -> Power Controllers/1(Q_abc)
  [Qset] -> Power Controllers/3(Q_set)
  [x_id] -> Converter State Deviation/2(x_id)
  [i_dq0] -> Converter State Deviation/1(i_dq0)
  Reference current limitation/3(||i_star_dq0_lim||) -> [i_star2_lim]
  [i_star_dq02_lim] -> Current Loop/1(i_star_dq0)
  [w_pll] -> Power Controllers/5(w_pll)
  [Pset] -> Converter State Deviation/3(pset)
  Pset/1 -> [Pset]
  [Pset] -> Power Controllers/6(P_set)
  Gain2/1 -> [i_abc]
  Three-Phase V-I Measurement/2 -> Memory11/1
  abc to dq3/1 -> [i_dq0]
  Memory10/1 -> [v_abc]
  Memory11/1 -> Gain2/1
  connections:
  i_dc1/LConn1 -- G_dc1/RConn1 -- Voltage Measurement/LConn2 -- Universal Bridge/RConn2 -- C_dc1/RConn1
  i_dc1/RConn1 -- G_dc1/LConn1 -- Voltage Measurement/LConn1 -- Universal Bridge/RConn1 -- C_dc1/LConn1
  RL Filter Element/RConn3 -- Universal Bridge/LConn3
  RL Filter Element/RConn2 -- Universal Bridge/LConn2
  RL Filter Element/RConn1 -- Universal Bridge/LConn1
  Three-Phase V-I Measurement/LConn1 -- RL Filter Element/LConn1
  Three-Phase V-I Measurement/LConn2 -- RL Filter Element/LConn2
  Three-Phase V-I Measurement/LConn3 -- RL Filter Element/LConn3
  Three-Phase V-I Measurement/RConn1 -- A/RConn1
  Three-Phase V-I Measurement/RConn2 -- B/RConn1
  Three-Phase V-I Measurement/RConn3 -- C/RConn1
